simulink model "CanInputInterface"  (R2019b)
settings: Solver=FixedStepAuto  StartTime=0.0  StopTime=10.0  RelTol=1e-3
undefined symbols (not defined in the file): MotorStates_e
libraries: simulink x1
settings Model: DataDictionary=CanInputInterface.sldd  Creator=unix  LastModifiedBy=unix

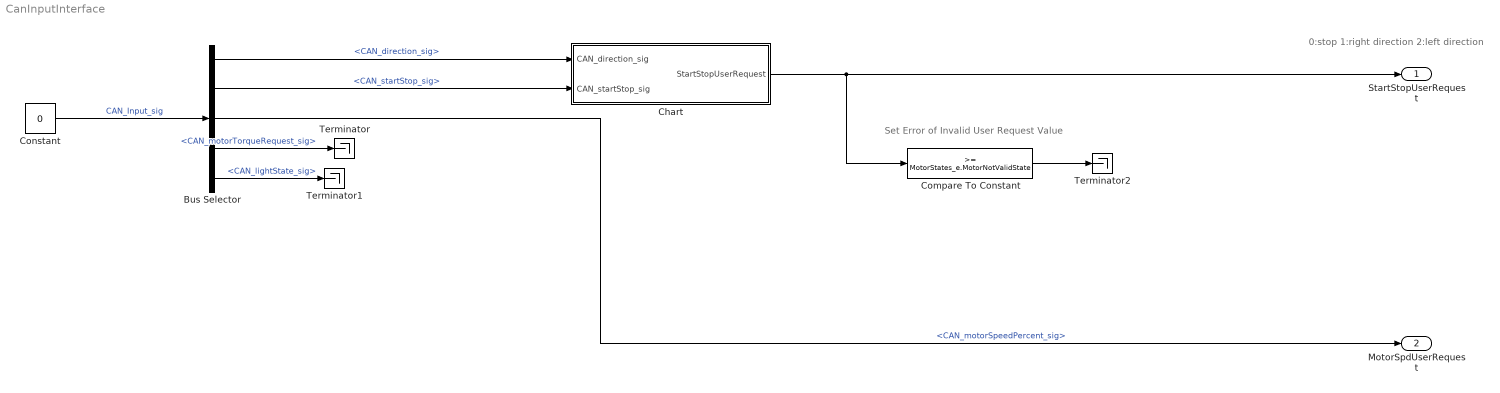
== system CanInputInterface ==
  note: Set Error of Invalid User Request Value
  note: 0:stop 1:right direction 2:left direction
  Bus Selector : BusSelector  OutputSignals=CAN_direction_sig,CAN_startStop_sig,CAN_motorSpeedPercent_sig,CAN_motorTorqueRequest_sig,CAN_lightState_sig
  Chart : Stateflow chart  BlockKeywords=__PRM__SERIALIZED__DATA__:Stateflow Chart,Stateflow Diagram  TreatAsAtomicUnit=on
  Compare To Constant : simulink/Logic and Bit Operations/Compare To Constant  relop=>=  const=MotorStates_e.MotorNotValidState  OutDataTypeStr=boolean
  Constant : Constant  Value=0  OutDataTypeStr=Bus: CAN_MotorCommands
  Terminator : Terminator
  Terminator1 : Terminator
  Terminator2 : Terminator
  StartStopUserRequest : Outport  OutDataTypeStr=Enum: MotorStates_e
  MotorSpdUserRequest : Outport  Port=2
  wires:
  Constant/1 -> Bus Selector/1  "CAN_Input_sig"
  Bus Selector/1 -> Chart/1(CAN_direction_sig)  "<CAN_direction_sig>"
  Bus Selector/2 -> Chart/2(CAN_startStop_sig)  "<CAN_startStop_sig>"
  Bus Selector/3 -> MotorSpdUserRequest/1  "<CAN_motorSpeedPercent_sig>"
  Bus Selector/4 -> Terminator/1  "<CAN_motorTorqueRequest_sig>"
  Bus Selector/5 -> Terminator1/1  "<CAN_lightState_sig>"
  Chart/1(StartStopUserRequest) -> Compare To Constant/1, StartStopUserRequest/1
  Compare To Constant/1 -> Terminator2/1

== stateflow chart CanInputInterface/Chart ==
  note: % ErrorCondition
  (default) -> (junction 22) : % MotorDirection
  (junction 22) -> (junction 23) [order 1] : [CAN_startStop_sig==0]
  (junction 22) -> (junction 24) [order 2]
  (junction 23) -> (junction 31) : {StartStopUserRequest=MotorStates_e.MotorStopped}
  (junction 24) -> (junction 25) [order 1] : [CAN_startStop_sig==1 && CAN_direction_sig==0 ]
  (junction 24) -> (junction 26) [order 2]
  (junction 25) -> (junction 30) : {StartStopUserRequest=MotorStates_e.MotorRightSpin}
  (junction 26) -> (junction 27) [order 1] : [CAN_startStop_sig==1 && CAN_direction_sig==1 ]
  (junction 26) -> (junction 28) [order 2] : {StartStopUserRequest=MotorStates_e.MotorNotValidState}
  (junction 27) -> (junction 29) : {StartStopUserRequest=MotorLeftSpin}
  (junction 29) -> (junction 28)
  (junction 30) -> (junction 29)
  (junction 31) -> (junction 30)
  (junction 28) -> (junction 32)
  data: CAN_direction_sig input; CAN_startStop_sig input; StartStopUserRequest output
